simulink model "rgb_gauss_sobel_64bit_full"  (R2022a)
settings: Solver=VariableStepAuto  StartTime=0.0  StopTime=10.0  RelTol=1e-3
values from neighbouring files (symbols this model uses):
  blueMax = 255    [setup.m]
  blueMin = 75    [setup.m]
  greenMax = 255    [setup.m]
  greenMin = 75    [setup.m]
  R = 752    [setup.m]
  redMax = 255    [setup.m]
  redMin = 75    [setup.m]
undefined symbols (not defined in the file or in its folder): gray
libraries: hdlsllib x64, visionhdlio x6, visionsources x2
settings Model: PacingRate=1000  Creator=cxc1831  LastModifiedBy=calvi
settings OptimizationCC: BlockReduction=off  ConditionallyExecuteInputs=off

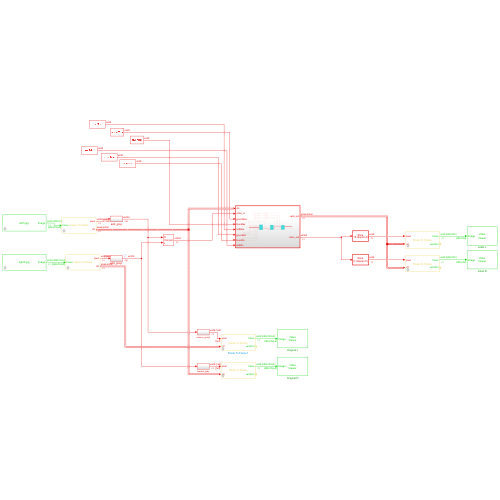
[thumbnail: Simulink's stored preview of the top-level diagram]
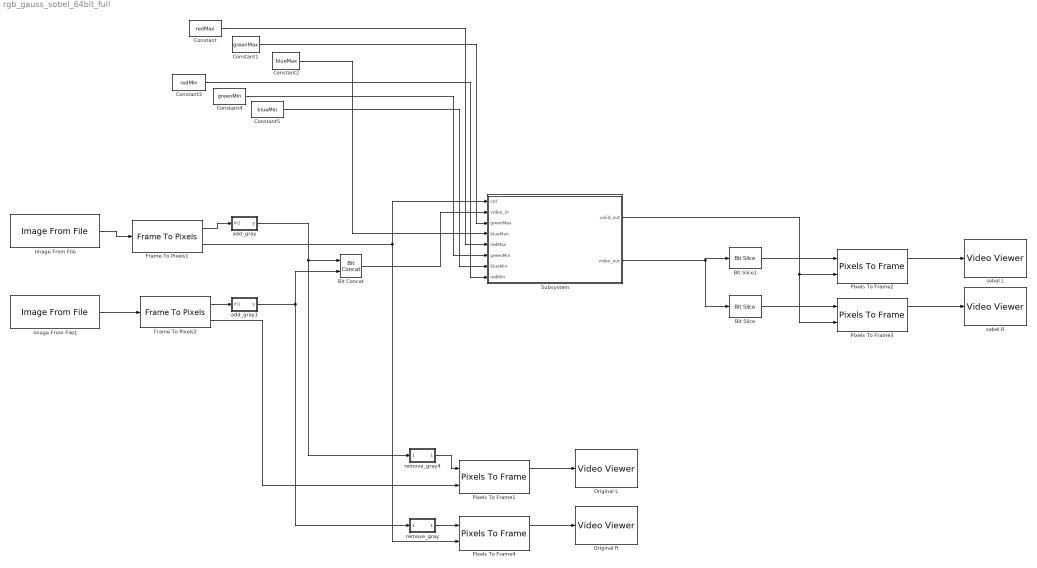
== system rgb_gauss_sobel_64bit_full ==
  Bit Concat : hdlsllib/Logic and Bit Operations/Bit Concat  numInputs=2
  Bit Slice : hdlsllib/Logic and Bit Operations/Bit Slice  lidx=7  ridx=0
      settings: SourceProductBaseCode=SL
  Bit Slice1 : hdlsllib/Logic and Bit Operations/Bit Slice  lidx=15  ridx=8
      settings: SourceProductBaseCode=SL
  Constant : Constant  Value=redMax  OutDataTypeStr=uint8  SampleTime=-1
  Constant1 : Constant  Value=greenMax  OutDataTypeStr=uint8  SampleTime=-1
  Constant2 : Constant  Value=blueMax  OutDataTypeStr=uint8  SampleTime=-1
  Constant3 : Constant  Value=redMin  OutDataTypeStr=uint8  SampleTime=-1  LockScale=on
  Constant4 : Constant  Value=greenMin  OutDataTypeStr=uint8  SampleTime=-1  LockScale=on
  Constant5 : Constant  Value=blueMin  OutDataTypeStr=uint8  SampleTime=-1  LockScale=on
  Frame To Pixels1 : visionhdlio/Frame To Pixels  NumComponents=3  NumPixels=1  VideoFormat=Custom  ActivePixelsPerLine=R  ActiveVideoLines=C  TotalPixelsPerLine=R  TotalVideoLines=C  StartingActiveLine=1  FrontPorch=0  SampleTime=0  VideoFormatCache=Custom  ActivePixelsPerLineCache=R  ActiveVideoLinesCache=C  TotalPixelsPerLineCache=R  TotalVideoLinesCache=C  StartingActiveLineCache=1  FrontPorchCache=0
      settings: SourceProductBaseCode=VT
  Frame To Pixels2 : visionhdlio/Frame To Pixels  NumComponents=3  NumPixels=1  VideoFormat=Custom  ActivePixelsPerLine=R  ActiveVideoLines=C  TotalPixelsPerLine=R  TotalVideoLines=C  StartingActiveLine=1  FrontPorch=0  SampleTime=0  VideoFormatCache=Custom  ActivePixelsPerLineCache=R  ActiveVideoLinesCache=C  TotalPixelsPerLineCache=R  TotalVideoLinesCache=C  StartingActiveLineCache=1  FrontPorchCache=0
      settings: SourceProductBaseCode=VT
  Image From File : visionsources/Image From File  Tag=vipblks_nd  FileName=C:\Projects\ipcore_integration\left3.jpg  Ts=1  imagePorts=One multidimensional signal  OutPortLabels=R|G|B  ImageDataType=Inherit from input image  sdImageDataType=uint(8)  Signed=on  WordLength=16  FractionLengthMode=User-defined  FractionLength=15
  Image From File1 : visionsources/Image From File  Tag=vipblks_nd  FileName=C:\Projects\ipcore_integration\right3.jpg  Ts=1  imagePorts=One multidimensional signal  OutPortLabels=R|G|B  ImageDataType=Inherit from input image  sdImageDataType=uint(8)  Signed=on  WordLength=16  FractionLengthMode=User-defined  FractionLength=15
  Original L : VideoViewer  colormapValue=gray(256)  FigPos=[1016 1123 562 322]
  Original R : VideoViewer  colormapValue=gray(256)  FigPos=[1046 1109 485 298]
  Pixels To Frame1 : visionhdlio/Pixels To Frame  NumComponents=3  NumPixels=1  VideoFormat=Custom  ActivePixelsPerLine=R  ActiveVideoLines=C  TotalPixelsPerLine=R  TotalVideoLines=C  VideoFormatCache=Custom  ActivePixelsPerLineCache=R  ActiveVideoLinesCache=C  TotalPixelsPerLineCache=R  TotalVideoLinesCache=C
      settings: SourceProductBaseCode=VT
  Pixels To Frame2 : visionhdlio/Pixels To Frame  NumComponents=1  NumPixels=1  VideoFormat=Custom  ActivePixelsPerLine=R  ActiveVideoLines=C  TotalPixelsPerLine=R  TotalVideoLines=C  VideoFormatCache=Custom  ActivePixelsPerLineCache=R  ActiveVideoLinesCache=C  TotalPixelsPerLineCache=R  TotalVideoLinesCache=C
      settings: SourceProductBaseCode=VT
  Pixels To Frame3 : visionhdlio/Pixels To Frame  NumComponents=1  NumPixels=1  VideoFormat=Custom  ActivePixelsPerLine=R  ActiveVideoLines=C  TotalPixelsPerLine=R  TotalVideoLines=C  VideoFormatCache=Custom  ActivePixelsPerLineCache=R  ActiveVideoLinesCache=C  TotalPixelsPerLineCache=R  TotalVideoLinesCache=C
      settings: SourceProductBaseCode=VT
  Pixels To Frame4 : visionhdlio/Pixels To Frame  NumComponents=3  NumPixels=1  VideoFormat=Custom  ActivePixelsPerLine=R  ActiveVideoLines=C  TotalPixelsPerLine=R  TotalVideoLines=C  VideoFormatCache=Custom  ActivePixelsPerLineCache=R  ActiveVideoLinesCache=C  TotalPixelsPerLineCache=R  TotalVideoLinesCache=C
      settings: SourceProductBaseCode=VT
  Subsystem : Subsystem  TreatAsAtomicUnit=on
  add_gray : Subsystem
  add_gray1 : Subsystem
  remove_gray : Subsystem
  remove_gray4 : Subsystem
  sobel L : VideoViewer  colormapValue=gray(256)  FigPos=[1 1398 2560 1298]
  sobel R : VideoViewer  colormapValue=gray(256)  FigPos=[1 1398 2560 1298]
  wires:
  Frame To Pixels2/2 -> Pixels To Frame1/2
  remove_gray4/1(RGBVector) -> Pixels To Frame1/1
  add_gray/1(y) -> remove_gray4/1(RGB), Bit Concat/1
  Image From File1/1 -> Frame To Pixels2/1
  remove_gray/1(RGBVector) -> Pixels To Frame4/1
  Frame To Pixels1/2 -> Subsystem/1(ctrl), Pixels To Frame4/2
  add_gray1/1(y) -> remove_gray/1(RGB), Bit Concat/2
  Image From File/1 -> Frame To Pixels1/1
  Frame To Pixels1/1 -> add_gray/1(In1)
  Frame To Pixels2/1 -> add_gray1/1(In1)
  Pixels To Frame1/1 -> Original L/1
  Pixels To Frame4/1 -> Original R/1
  Pixels To Frame2/1 -> sobel L/1
  Pixels To Frame3/1 -> sobel R/1
  Bit Slice/1 -> Pixels To Frame3/1
  Bit Slice1/1 -> Pixels To Frame2/1
  Bit Concat/1 -> Subsystem/2(video_in)
  Subsystem/2(video_out) -> Bit Slice1/1, Bit Slice/1
  Subsystem/1(valid_out) -> Pixels To Frame3/2, Pixels To Frame2/2
  Constant1/1 -> Subsystem/3(greenMax)
  Constant/1 -> Subsystem/5(redMax)
  Constant2/1 -> Subsystem/4(blueMax)
  Constant3/1 -> Subsystem/8(redMin)
  Constant4/1 -> Subsystem/6(greenMin)
  Constant5/1 -> Subsystem/7(blueMin)

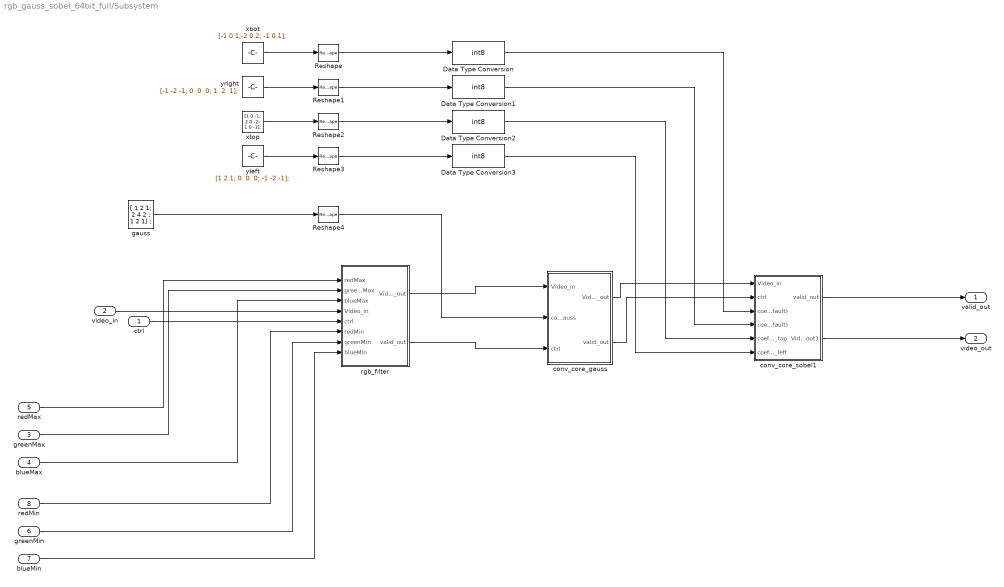
== system rgb_gauss_sobel_64bit_full/Subsystem ==
  ctrl : Inport
  video_in : Inport  Port=2
  greenMax : Inport  Port=3
  blueMax : Inport  Port=4
  redMax : Inport  Port=5
  greenMin : Inport  Port=6
  blueMin : Inport  Port=7
  redMin : Inport  Port=8
  Data Type Conversion{,1..3} (4 alike) : DataTypeConversion  OutDataTypeStr=int8  SaturateOnIntegerOverflow=off  RndMeth=Floor
  Reshape{,1..4} (5 alike) : Reshape
  conv_core_gauss : Subsystem  TreatAsAtomicUnit=on
  conv_core_sobel1 : Subsystem  TreatAsAtomicUnit=on
  gauss : Constant  Value=|  VectorParams1D=off  OutDataTypeStr=uint8  SampleTime=-1  LockScale=on
      | [ 1  2  1;  2   4   2 ;  1  2  1]
      | ;
  rgb_filter : Subsystem  TreatAsAtomicUnit=on
  xbot : Constant  Value=|  VectorParams1D=off  OutDataTypeStr=int8  SampleTime=-1
      | [-1 0 1;-2 0 2;
      | -1 0 1];
  xtop : Constant  Value=|  VectorParams1D=off  OutDataTypeStr=int8  SampleTime=-1
      | [1 0 -1; 2 0 -2;
      | 1 0 -1];
  yleft : Constant  Value="[1 2 1; 0  0  0; -1 -2 -1];"  VectorParams1D=off  OutDataTypeStr=int8  SampleTime=-1
  yright : Constant  Value=|  VectorParams1D=off  OutDataTypeStr=int8  SampleTime=-1
      | [-1 -2 -1;
      | 0  0  0; 1  2  1];
  valid_out : Outport
  video_out : Outport  Port=2
  wires:
  xtop/1 -> Reshape2/1
  yleft/1 -> Reshape3/1
  conv_core_sobel1/2(Video_out1) -> video_out/1
  xbot/1 -> Reshape/1
  yright/1 -> Reshape1/1
  conv_core_sobel1/1(valid_out) -> valid_out/1
  Reshape/1 -> Data Type Conversion/1
  Reshape1/1 -> Data Type Conversion1/1
  Reshape2/1 -> Data Type Conversion2/1
  Reshape3/1 -> Data Type Conversion3/1
  Data Type Conversion/1 -> conv_core_sobel1/3(coeffsX_bot(default))
  Data Type Conversion1/1 -> conv_core_sobel1/4(coeffsY_right(default))
  Data Type Conversion2/1 -> conv_core_sobel1/5(coeffsX_top)
  Data Type Conversion3/1 -> conv_core_sobel1/6(coeffsY_left)
  Reshape4/1 -> conv_core_gauss/2(coeffsGauss)
  gauss/1 -> Reshape4/1
  greenMin/1 -> rgb_filter/7(greenMin)
  redMax/1 -> rgb_filter/1(redMax)
  redMin/1 -> rgb_filter/6(redMin)
  greenMax/1 -> rgb_filter/2(greenMax)
  blueMax/1 -> rgb_filter/3(blueMax)
  blueMin/1 -> rgb_filter/8(blueMin)
  ctrl/1 -> rgb_filter/5(ctrl)
  video_in/1 -> rgb_filter/4(Video_in)
  rgb_filter/1(Video_out) -> conv_core_gauss/1(Video_in)
  rgb_filter/2(valid_out) -> conv_core_gauss/3(ctrl)
  conv_core_gauss/1(Video_out) -> conv_core_sobel1/1(Video_in)
  conv_core_gauss/2(valid_out) -> conv_core_sobel1/2(ctrl)

== system rgb_gauss_sobel_64bit_full/add_gray ==
  note: Grayscale = (R * 0.25) + (G * 0.5) + (B * 0.125)
  In1 : Inport
  Bit Concat : hdlsllib/Logic and Bit Operations/Bit Concat  numInputs=4
  Demux : Demux  Outputs=3
  Shift Arithmetic3 : ArithShift  BitShiftNumber=1  BitShiftDirection=Right
  Shift Arithmetic4 : ArithShift  BitShiftNumber=2  BitShiftDirection=Right
  Shift Arithmetic5 : ArithShift  BitShiftNumber=3  BitShiftDirection=Right
  Sum : Sum  Inputs=+++  OutDataTypeStr=uint8
  y : Outport
  wires:
  Bit Concat/1 -> y/1
  In1/1 -> Demux/1
  Demux/2 -> Shift Arithmetic3/1, Bit Concat/3
  Demux/1 -> Shift Arithmetic4/1, Bit Concat/2
  Demux/3 -> Shift Arithmetic5/1, Bit Concat/4
  Sum/1 -> Bit Concat/1
  Shift Arithmetic4/1 -> Sum/1
  Shift Arithmetic3/1 -> Sum/2
  Shift Arithmetic5/1 -> Sum/3

== system rgb_gauss_sobel_64bit_full/add_gray1 ==
  note: Grayscale = (R * 0.25) + (G * 0.5) + (B * 0.125)
  In1 : Inport
  Bit Concat : hdlsllib/Logic and Bit Operations/Bit Concat  numInputs=4
  Demux : Demux  Outputs=3
  Shift Arithmetic3 : ArithShift  BitShiftNumber=1  BitShiftDirection=Right
  Shift Arithmetic4 : ArithShift  BitShiftNumber=2  BitShiftDirection=Right
  Shift Arithmetic5 : ArithShift  BitShiftNumber=3  BitShiftDirection=Right
  Sum : Sum  Inputs=+++  OutDataTypeStr=uint8
  y : Outport
  wires:
  Bit Concat/1 -> y/1
  In1/1 -> Demux/1
  Demux/2 -> Shift Arithmetic3/1, Bit Concat/3
  Demux/1 -> Shift Arithmetic4/1, Bit Concat/2
  Demux/3 -> Shift Arithmetic5/1, Bit Concat/4
  Sum/1 -> Bit Concat/1
  Shift Arithmetic4/1 -> Sum/1
  Shift Arithmetic3/1 -> Sum/2
  Shift Arithmetic5/1 -> Sum/3

== system rgb_gauss_sobel_64bit_full/remove_gray ==
  note: RGB represented in
      | 32'hFFRRGGBB
  RGB : Inport
  Bit Slice : hdlsllib/Logic and Bit Operations/Bit Slice  lidx=23  ridx=16
      settings: SourceProductBaseCode=SL
  Bit Slice1 : hdlsllib/Logic and Bit Operations/Bit Slice  lidx=15  ridx=8
      settings: SourceProductBaseCode=SL
  Bit Slice2 : hdlsllib/Logic and Bit Operations/Bit Slice  lidx=7  ridx=0
      settings: SourceProductBaseCode=SL
  Mux : Mux  Inputs=3
  Signal Specification : SignalSpecification
  Transpose : Math  Operator=transpose  SignedPower=on
  RGBVector : Outport  VectorParamsAs1DForOutWhenUnconnected=off
  wires:
  Signal Specification/1 -> RGBVector/1
  Transpose/1 -> Signal Specification/1
  RGB/1 -> Bit Slice/1, Bit Slice1/1, Bit Slice2/1
  Bit Slice1/1 -> Mux/2
  Bit Slice2/1 -> Mux/3
  Bit Slice/1 -> Mux/1
  Mux/1 -> Transpose/1

== system rgb_gauss_sobel_64bit_full/remove_gray4 ==
  note: RGB represented in
      | 32'hFFRRGGBB
  RGB : Inport
  Bit Slice : hdlsllib/Logic and Bit Operations/Bit Slice  lidx=23  ridx=16
      settings: SourceProductBaseCode=SL
  Bit Slice1 : hdlsllib/Logic and Bit Operations/Bit Slice  lidx=15  ridx=8
      settings: SourceProductBaseCode=SL
  Bit Slice2 : hdlsllib/Logic and Bit Operations/Bit Slice  lidx=7  ridx=0
      settings: SourceProductBaseCode=SL
  Mux : Mux  Inputs=3
  Signal Specification : SignalSpecification
  Transpose : Math  Operator=transpose  SignedPower=on
  RGBVector : Outport  VectorParamsAs1DForOutWhenUnconnected=off
  wires:
  Signal Specification/1 -> RGBVector/1
  Transpose/1 -> Signal Specification/1
  RGB/1 -> Bit Slice/1, Bit Slice1/1, Bit Slice2/1
  Bit Slice1/1 -> Mux/2
  Bit Slice2/1 -> Mux/3
  Bit Slice/1 -> Mux/1
  Mux/1 -> Transpose/1

== system rgb_gauss_sobel_64bit_full/Subsystem/conv_core_gauss ==
  Video_in : Inport
  coeffsGauss : Inport  Port=2
  ctrl : Inport  Port=3
  Bus Selector : BusSelector  OutputSignals=valid
  Delay1 : Delay  InitialCondition=0
  Subsystem1 : Subsystem
  Video_out : Outport  VectorParamsAs1DForOutWhenUnconnected=off
  valid_out : Outport  Port=2  VectorParamsAs1DForOutWhenUnconnected=off
  wires:
  Video_in/1 -> Subsystem1/1(VideoIn)
  ctrl/1 -> Bus Selector/1, Delay1/1
  Bus Selector/1 -> Subsystem1/Enable  "<valid>"
  Subsystem1/1(Video_out) -> Video_out/1
  Delay1/1 -> valid_out/1
  coeffsGauss/1 -> Subsystem1/2(coeffsGauss)

== system rgb_gauss_sobel_64bit_full/Subsystem/conv_core_sobel1 ==
  Video_in : Inport
  ctrl : Inport  Port=2
  coeffsX_bot(default) : Inport  Port=3
  coeffsY_right(default) : Inport  Port=4
  coeffsX_top : Inport  Port=5
  coeffsY_left : Inport  Port=6
  Bit Concat1 : hdlsllib/Logic and Bit Operations/Bit Concat  numInputs=2
  Bus Selector : BusSelector  OutputSignals=valid
  Delay1 : Delay  InitialCondition=0
  Subsystem1 : Subsystem
  valid_out : Outport  VectorParamsAs1DForOutWhenUnconnected=off
  Video_out1 : Outport  Port=2  VectorParamsAs1DForOutWhenUnconnected=off
  wires:
  Video_in/1 -> Subsystem1/1(vidIn)
  ctrl/1 -> Bus Selector/1, Subsystem1/4(ctrl), Delay1/1
  Bus Selector/1 -> Subsystem1/Enable  "<valid>"
  Delay1/1 -> valid_out/1
  coeffsY_right(default)/1 -> Subsystem1/3(coeffsY_bot(default))
  coeffsX_bot(default)/1 -> Subsystem1/2(coeffsX_bot(default))
  Bit Concat1/1 -> Video_out1/1
  Subsystem1/1(sobel R) -> Bit Concat1/2
  Subsystem1/2(sobel L) -> Bit Concat1/1
  coeffsX_top/1 -> Subsystem1/5(coeffsX_Top)
  coeffsY_left/1 -> Subsystem1/6(coeffsY_Left)

== system rgb_gauss_sobel_64bit_full/Subsystem/rgb_filter ==
  redMax : Inport
  greenMax : Inport  Port=2
  blueMax : Inport  Port=3
  Video_in : Inport  Port=4
  ctrl : Inport  Port=5
  redMin : Inport  Port=6  OutDataTypeStr=uint8
  greenMin : Inport  Port=7  OutDataTypeStr=uint8
  blueMin : Inport  Port=8  OutDataTypeStr=uint8
  Bit Concat1 : hdlsllib/Logic and Bit Operations/Bit Concat  numInputs=2
  Bus Selector : BusSelector  OutputSignals=valid
  Delay1 : Delay  DelayLength=1  InitialCondition=0
  Subsystem1 : Subsystem
  Video_out : Outport  VectorParamsAs1DForOutWhenUnconnected=off
  valid_out : Outport  Port=2  VectorParamsAs1DForOutWhenUnconnected=off
  wires:
  Video_in/1 -> Subsystem1/1(In2)
  ctrl/1 -> Bus Selector/1, Delay1/1
  Bus Selector/1 -> Subsystem1/Enable  "<valid>"
  redMax/1 -> Subsystem1/2(redmax)
  Delay1/1 -> valid_out/1
  greenMax/1 -> Subsystem1/3(greenmax)
  blueMax/1 -> Subsystem1/4(bluemax)
  Bit Concat1/1 -> Video_out/1
  redMin/1 -> Subsystem1/5(redMin)
  Subsystem1/2(Video_outRight) -> Bit Concat1/2
  Subsystem1/1(Video_outLeft) -> Bit Concat1/1
  greenMin/1 -> Subsystem1/6(greenMin)
  blueMin/1 -> Subsystem1/7(blueMin)

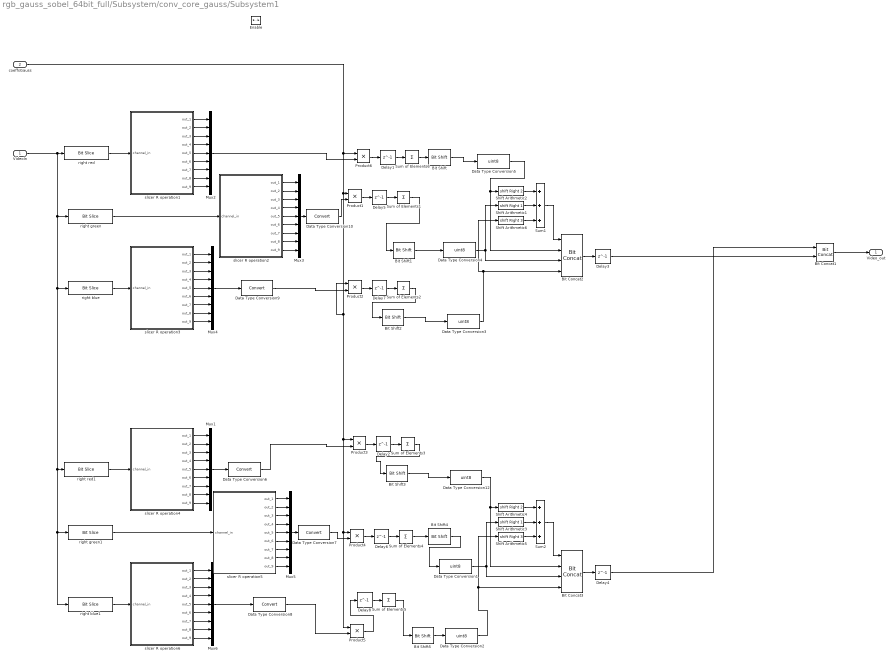
== system rgb_gauss_sobel_64bit_full/Subsystem/conv_core_gauss/Subsystem1 ==
  VideoIn : Inport
  coeffsGauss : Inport  Port=2
  Enable : EnablePort
  Bit Concat1 : hdlsllib/Logic and Bit Operations/Bit Concat  numInputs=2
  Bit Concat2 : hdlsllib/Logic and Bit Operations/Bit Concat  numInputs=4
  Bit Concat3 : hdlsllib/Logic and Bit Operations/Bit Concat  numInputs=4
  Bit Shift{,1..5} (6 alike) : hdlsllib/Logic and Bit Operations/Bit Shift  mode=Shift Right Arithmetic  N=4
  Data Type Conversion{1..5,12} (6 alike) : DataTypeConversion  OutDataTypeStr=uint8  SaturateOnIntegerOverflow=off  RndMeth=Floor
  Data Type Conversion{6..10} (5 alike) : DataTypeConversion  SaturateOnIntegerOverflow=off  RndMeth=Floor
  Delay{1..8} (8 alike) : Delay  DelayLength=1  InitialCondition=0
  Mux{1..6} (6 alike) : Mux  Inputs=9
  Product{1..6} (6 alike) : Product  SaturateOnIntegerOverflow=on
  Shift Arithmetic1 : ArithShift  BitShiftNumber=1  BitShiftDirection=Right
  Shift Arithmetic2 : ArithShift  BitShiftNumber=2  BitShiftDirection=Right
  Shift Arithmetic3 : ArithShift  BitShiftNumber=1  BitShiftDirection=Right
  Shift Arithmetic4 : ArithShift  BitShiftNumber=2  BitShiftDirection=Right
  Shift Arithmetic5 : ArithShift  BitShiftNumber=3  BitShiftDirection=Right
  Shift Arithmetic6 : ArithShift  BitShiftNumber=3  BitShiftDirection=Right
  Sum of Elements{1..6} (6 alike) : Sum  Inputs=+  OutDataTypeStr=uint32  SaturateOnIntegerOverflow=on
  Sum1 : Sum  Inputs=+++  OutDataTypeStr=uint8
  Sum2 : Sum  Inputs=+++  OutDataTypeStr=uint8
  right blue : hdlsllib/Logic and Bit Operations/Bit Slice  lidx=7  ridx=0
      settings: SourceProductBaseCode=SL
  right blue1 : hdlsllib/Logic and Bit Operations/Bit Slice  lidx=39  ridx=32
      settings: SourceProductBaseCode=SL
  right green : hdlsllib/Logic and Bit Operations/Bit Slice  lidx=15  ridx=8
      settings: SourceProductBaseCode=SL
  right green1 : hdlsllib/Logic and Bit Operations/Bit Slice  lidx=47  ridx=40
      settings: SourceProductBaseCode=SL
  right red : hdlsllib/Logic and Bit Operations/Bit Slice  lidx=23  ridx=16
      settings: SourceProductBaseCode=SL
  right red1 : hdlsllib/Logic and Bit Operations/Bit Slice  lidx=55  ridx=48
      settings: SourceProductBaseCode=SL
  slicer R operation1 : Subsystem
  slicer R operation2 : Subsystem
  slicer R operation3 : Subsystem
  slicer R operation4 : Subsystem
  slicer R operation5 : Subsystem
  slicer R operation6 : Subsystem
  Video_out : Outport  InitialOutput=0  VectorParamsAs1DForOutWhenUnconnected=off
  wires:
  right red/1 -> slicer R operation1/1(channel_in)
  right green/1 -> slicer R operation2/1(channel_in)
  right blue/1 -> slicer R operation3/1(channel_in)
  slicer R operation1/4(out_4) -> Mux2/4
  slicer R operation1/9(out_9) -> Mux2/9
  slicer R operation1/7(out_7) -> Mux2/7
  slicer R operation1/1(out_1) -> Mux2/1
  slicer R operation1/5(out_5) -> Mux2/5
  slicer R operation1/6(out_6) -> Mux2/6
  slicer R operation1/3(out_3) -> Mux2/3
  slicer R operation1/8(out_8) -> Mux2/8
  slicer R operation1/2(out_2) -> Mux2/2
  slicer R operation2/4(out_4) -> Mux3/4
  slicer R operation2/9(out_9) -> Mux3/9
  slicer R operation2/7(out_7) -> Mux3/7
  slicer R operation2/1(out_1) -> Mux3/1
  slicer R operation2/5(out_5) -> Mux3/5
  slicer R operation2/6(out_6) -> Mux3/6
  slicer R operation2/3(out_3) -> Mux3/3
  slicer R operation2/8(out_8) -> Mux3/8
  slicer R operation2/2(out_2) -> Mux3/2
  slicer R operation3/4(out_4) -> Mux4/4
  slicer R operation3/9(out_9) -> Mux4/9
  slicer R operation3/7(out_7) -> Mux4/7
  slicer R operation3/1(out_1) -> Mux4/1
  slicer R operation3/5(out_5) -> Mux4/5
  slicer R operation3/6(out_6) -> Mux4/6
  slicer R operation3/3(out_3) -> Mux4/3
  slicer R operation3/8(out_8) -> Mux4/8
  slicer R operation3/2(out_2) -> Mux4/2
  Product1/1 -> Delay5/1
  Mux3/1 -> Data Type Conversion10/1
  Mux4/1 -> Data Type Conversion9/1
  Data Type Conversion3/1 -> Shift Arithmetic6/1, Bit Concat2/4
  Sum of Elements1/1 -> Bit Shift1/1
  Data Type Conversion5/1 -> Bit Concat2/2, Shift Arithmetic2/1
  Bit Concat2/1 -> Delay3/1
  Shift Arithmetic1/1 -> Sum1/2
  Shift Arithmetic2/1 -> Sum1/1
  Shift Arithmetic6/1 -> Sum1/3
  Sum1/1 -> Bit Concat2/1
  Bit Concat1/1 -> Video_out/1
  Sum2/1 -> Bit Concat3/1
  right green1/1 -> slicer R operation5/1(channel_in)
  Shift Arithmetic4/1 -> Sum2/1
  Bit Concat3/1 -> Delay4/1
  slicer R operation4/5(out_5) -> Mux1/5
  Mux6/1 -> Data Type Conversion8/1
  Data Type Conversion12/1 -> Bit Concat3/2, Shift Arithmetic4/1
  slicer R operation6/1(out_1) -> Mux6/1
  slicer R operation4/9(out_9) -> Mux1/9
  slicer R operation6/3(out_3) -> Mux6/3
  slicer R operation6/5(out_5) -> Mux6/5
  Data Type Conversion2/1 -> Shift Arithmetic5/1, Bit Concat3/4
  slicer R operation6/9(out_9) -> Mux6/9
  slicer R operation6/8(out_8) -> Mux6/8
  slicer R operation6/4(out_4) -> Mux6/4
  right red1/1 -> slicer R operation4/1(channel_in)
  slicer R operation5/2(out_2) -> Mux5/2
  slicer R operation5/5(out_5) -> Mux5/5
  slicer R operation6/6(out_6) -> Mux6/6
  Mux1/1 -> Data Type Conversion6/1
  slicer R operation5/4(out_4) -> Mux5/4
  slicer R operation5/7(out_7) -> Mux5/7
  slicer R operation5/6(out_6) -> Mux5/6
  coeffsGauss/1 -> Product6/1, Product2/1, Product5/1, Product4/1, Product3/1, Product1/1
  slicer R operation4/7(out_7) -> Mux1/7
  slicer R operation4/3(out_3) -> Mux1/3
  slicer R operation6/7(out_7) -> Mux6/7
  slicer R operation5/3(out_3) -> Mux5/3
  Data Type Conversion1/1 -> Shift Arithmetic3/1, Bit Concat3/3
  slicer R operation5/1(out_1) -> Mux5/1
  slicer R operation5/9(out_9) -> Mux5/9
  slicer R operation4/1(out_1) -> Mux1/1
  slicer R operation4/2(out_2) -> Mux1/2
  right blue1/1 -> slicer R operation6/1(channel_in)
  slicer R operation5/8(out_8) -> Mux5/8
  Shift Arithmetic5/1 -> Sum2/3
  Shift Arithmetic3/1 -> Sum2/2
  slicer R operation6/2(out_2) -> Mux6/2
  slicer R operation4/4(out_4) -> Mux1/4
  slicer R operation4/8(out_8) -> Mux1/8
  VideoIn/1 -> right blue1/1, right green1/1, right red1/1, right blue/1, right green/1, right red/1
  slicer R operation4/6(out_6) -> Mux1/6
  Delay4/1 -> Bit Concat1/1
  Delay3/1 -> Bit Concat1/2
  Data Type Conversion6/1 -> Product3/2
  Mux5/1 -> Data Type Conversion7/1
  Data Type Conversion7/1 -> Product4/2
  Data Type Conversion8/1 -> Product5/2
  Data Type Conversion9/1 -> Product2/2
  Data Type Conversion10/1 -> Product1/2
  Mux2/1 -> Product6/2
  Bit Shift1/1 -> Data Type Conversion4/1
  Delay5/1 -> Sum of Elements1/1
  Data Type Conversion4/1 -> Bit Concat2/3, Shift Arithmetic1/1
  Bit Shift/1 -> Data Type Conversion5/1
  Sum of Elements6/1 -> Bit Shift/1
  Product6/1 -> Delay1/1
  Delay1/1 -> Sum of Elements6/1
  Bit Shift2/1 -> Data Type Conversion3/1
  Product2/1 -> Delay7/1
  Delay7/1 -> Sum of Elements2/1
  Bit Shift3/1 -> Data Type Conversion12/1
  Product3/1 -> Delay2/1
  Delay2/1 -> Sum of Elements3/1
  Bit Shift4/1 -> Data Type Conversion1/1
  Sum of Elements4/1 -> Bit Shift4/1
  Product4/1 -> Delay6/1
  Delay6/1 -> Sum of Elements4/1
  Bit Shift5/1 -> Data Type Conversion2/1
  Product5/1 -> Delay8/1
  Delay8/1 -> Sum of Elements5/1
  Sum of Elements2/1 -> Bit Shift2/1
  Sum of Elements3/1 -> Bit Shift3/1
  Sum of Elements5/1 -> Bit Shift5/1

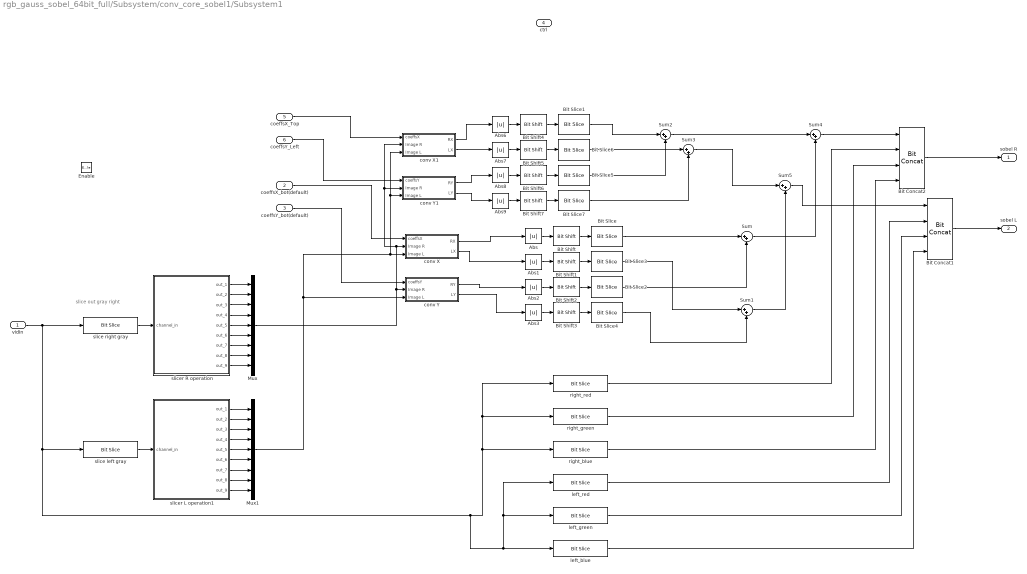
== system rgb_gauss_sobel_64bit_full/Subsystem/conv_core_sobel1/Subsystem1 ==
  note: slice out gray right
  vidIn : Inport
  coeffsX_bot(default) : Inport  Port=2
  coeffsY_bot(default) : Inport  Port=3
  ctrl : Inport  Port=4
  coeffsX_Top : Inport  Port=5
  coeffsY_Left : Inport  Port=6
  Enable : EnablePort
  Abs{,1..3,6..9} (8 alike) : Abs  SaturateOnIntegerOverflow=off
  Bit Concat1 : hdlsllib/Logic and Bit Operations/Bit Concat  numInputs=4
  Bit Concat2 : hdlsllib/Logic and Bit Operations/Bit Concat  numInputs=4
  Bit Shift{,1..7} (8 alike) : hdlsllib/Logic and Bit Operations/Bit Shift  mode=Shift Right Logical  N=1
  Bit Slice{,1..7} (8 alike) : hdlsllib/Logic and Bit Operations/Bit Slice  lidx=6  ridx=0
      settings: SourceProductBaseCode=SL
  Mux : Mux  Inputs=9
  Mux1 : Mux  Inputs=9
  Sum{,1..5} (6 alike) : Sum  Inputs=|++
  conv X : Subsystem
  conv X1 : Subsystem
  conv Y : Subsystem
  conv Y1 : Subsystem
  left_blue : hdlsllib/Logic and Bit Operations/Bit Slice  lidx=39  ridx=32
      settings: SourceProductBaseCode=SL
  left_green : hdlsllib/Logic and Bit Operations/Bit Slice  lidx=47  ridx=40
      settings: SourceProductBaseCode=SL
  left_red : hdlsllib/Logic and Bit Operations/Bit Slice  lidx=55  ridx=48
      settings: SourceProductBaseCode=SL
  right_blue : hdlsllib/Logic and Bit Operations/Bit Slice  lidx=7  ridx=0
      settings: SourceProductBaseCode=SL
  right_green : hdlsllib/Logic and Bit Operations/Bit Slice  lidx=15  ridx=8
      settings: SourceProductBaseCode=SL
  right_red : hdlsllib/Logic and Bit Operations/Bit Slice  lidx=23  ridx=16
      settings: SourceProductBaseCode=SL
  slice left gray : hdlsllib/Logic and Bit Operations/Bit Slice  lidx=63  ridx=56
      settings: SourceProductBaseCode=SL
  slice right gray : hdlsllib/Logic and Bit Operations/Bit Slice  lidx=31  ridx=24
      settings: SourceProductBaseCode=SL
  slicer L operation1 : Subsystem
  slicer R operation : Subsystem
  sobel R : Outport  InitialOutput=0
  sobel L : Outport  Port=2  InitialOutput=0
  wires:
  slicer R operation/1(out_1) -> Mux/1
  slicer R operation/9(out_9) -> Mux/9
  slicer R operation/5(out_5) -> Mux/5
  slicer R operation/7(out_7) -> Mux/7
  slicer R operation/3(out_3) -> Mux/3
  slicer R operation/6(out_6) -> Mux/6
  slicer R operation/4(out_4) -> Mux/4
  slicer R operation/2(out_2) -> Mux/2
  slicer R operation/8(out_8) -> Mux/8
  Mux/1 -> conv X/2(Image R), conv Y1/2(Image R), conv X1/2(Image R), conv Y/2(Image R)
  conv X/1(RX) -> Abs/1
  slice right gray/1 -> slicer R operation/1(channel_in)
  coeffsX_bot(default)/1 -> conv X/1(coeffsX)
  coeffsY_bot(default)/1 -> conv Y/1(coeffsY)
  slicer L operation1/9(out_9) -> Mux1/9
  slicer L operation1/8(out_8) -> Mux1/8
  slicer L operation1/6(out_6) -> Mux1/6
  slicer L operation1/5(out_5) -> Mux1/5
  slicer L operation1/3(out_3) -> Mux1/3
  slicer L operation1/2(out_2) -> Mux1/2
  slicer L operation1/7(out_7) -> Mux1/7
  slicer L operation1/4(out_4) -> Mux1/4
  slicer L operation1/1(out_1) -> Mux1/1
  slice left gray/1 -> slicer L operation1/1(channel_in)
  Mux1/1 -> conv Y/3(Image L), conv X1/3(Image L), conv Y1/3(Image L), conv X/3(Image L)
  conv Y/2(LY) -> Abs3/1
  conv X/2(LX) -> Abs1/1
  Bit Shift3/1 -> Bit Slice4/1
  Bit Shift2/1 -> Bit Slice2/1
  Bit Shift1/1 -> Bit Slice3/1
  Bit Shift/1 -> Bit Slice/1
  Bit Slice/1 -> Sum/1
  Bit Slice2/1 -> Sum/2
  Bit Slice3/1 -> Sum1/1
  Bit Slice4/1 -> Sum1/2
  conv Y/1(RY) -> Abs2/1
  Abs/1 -> Bit Shift/1
  Abs1/1 -> Bit Shift1/1
  Abs2/1 -> Bit Shift2/1
  Abs3/1 -> Bit Shift3/1
  Sum/1 -> Sum4/2
  coeffsX_Top/1 -> conv X1/1(coeffsX)
  coeffsY_Left/1 -> conv Y1/1(coeffsY)
  Bit Shift5/1 -> Bit Slice6/1
  Abs8/1 -> Bit Shift6/1
  Abs6/1 -> Bit Shift4/1
  Bit Shift6/1 -> Bit Slice5/1
  Abs9/1 -> Bit Shift7/1
  Bit Shift4/1 -> Bit Slice1/1
  Bit Shift7/1 -> Bit Slice7/1
  Abs7/1 -> Bit Shift5/1
  conv X1/1(RX) -> Abs6/1
  conv X1/2(LX) -> Abs7/1
  conv Y1/1(RY) -> Abs8/1
  conv Y1/2(LY) -> Abs9/1
  Sum2/1 -> Sum4/1
  Bit Slice1/1 -> Sum2/1
  Sum3/1 -> Sum5/1
  Sum1/1 -> Sum5/2
  Bit Slice5/1 -> Sum2/2
  Bit Slice6/1 -> Sum3/1
  Bit Slice7/1 -> Sum3/2
  vidIn/1 -> slice right gray/1, right_blue/1, right_green/1, right_red/1, left_red/1, left_green/1, left_blue/1, slice left gray/1
  Sum4/1 -> Bit Concat2/1
  Bit Concat2/1 -> sobel R/1
  right_red/1 -> Bit Concat2/2
  right_green/1 -> Bit Concat2/3
  right_blue/1 -> Bit Concat2/4
  Bit Concat1/1 -> sobel L/1
  left_blue/1 -> Bit Concat1/4
  left_green/1 -> Bit Concat1/3
  left_red/1 -> Bit Concat1/2
  Sum5/1 -> Bit Concat1/1

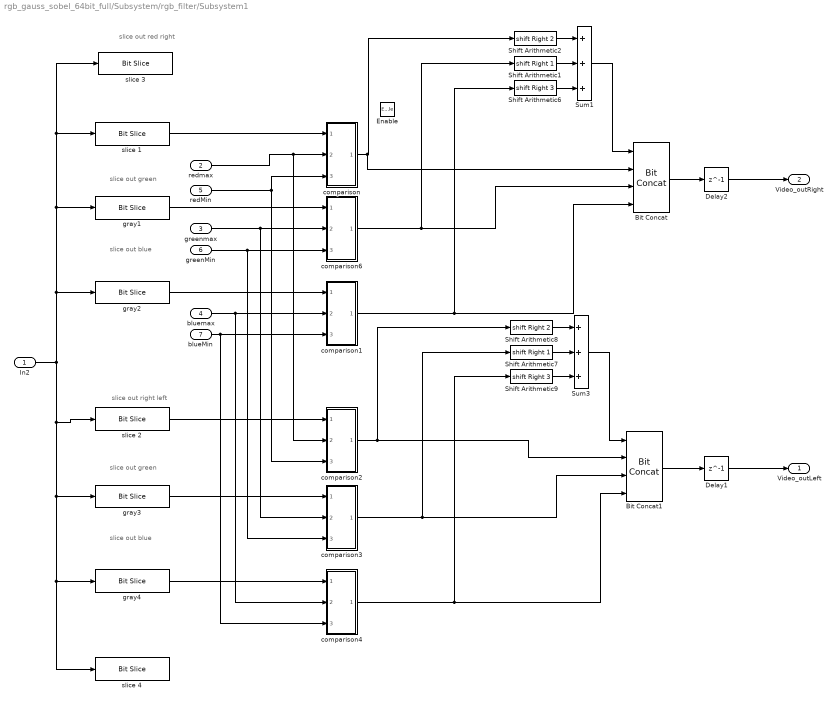
== system rgb_gauss_sobel_64bit_full/Subsystem/rgb_filter/Subsystem1 ==
  note: slice out red right
  note: slice out green
  note: slice out blue
  note: slice out blue
  note: slice out right left
  note: slice out green
  In2 : Inport
  redmax : Inport  Port=2
  greenmax : Inport  Port=3
  bluemax : Inport  Port=4
  redMin : Inport  Port=5  OutDataTypeStr=uint8
  greenMin : Inport  Port=6  OutDataTypeStr=uint8
  blueMin : Inport  Port=7  OutDataTypeStr=uint8
  Enable : EnablePort
  Bit Concat : hdlsllib/Logic and Bit Operations/Bit Concat  numInputs=4
  Bit Concat1 : hdlsllib/Logic and Bit Operations/Bit Concat  numInputs=4
  Delay1 : Delay  DelayLength=1  InitialCondition=0
  Delay2 : Delay  DelayLength=1  InitialCondition=0
  Shift Arithmetic1 : ArithShift  BitShiftNumber=1  BitShiftDirection=Right
  Shift Arithmetic2 : ArithShift  BitShiftNumber=2  BitShiftDirection=Right
  Shift Arithmetic6 : ArithShift  BitShiftNumber=3  BitShiftDirection=Right
  Shift Arithmetic7 : ArithShift  BitShiftNumber=1  BitShiftDirection=Right
  Shift Arithmetic8 : ArithShift  BitShiftNumber=2  BitShiftDirection=Right
  Shift Arithmetic9 : ArithShift  BitShiftNumber=3  BitShiftDirection=Right
  Sum1 : Sum  Inputs=+++  OutDataTypeStr=uint8
  Sum3 : Sum  Inputs=+++  OutDataTypeStr=uint8
  comparison : Subsystem
  comparison1 : Subsystem
  comparison2 : Subsystem
  comparison3 : Subsystem
  comparison4 : Subsystem
  comparison6 : Subsystem
  gray1 : hdlsllib/Logic and Bit Operations/Bit Slice  lidx=15  ridx=8
      settings: SourceProductBaseCode=SL
  gray2 : hdlsllib/Logic and Bit Operations/Bit Slice  lidx=7  ridx=0
      settings: SourceProductBaseCode=SL
  gray3 : hdlsllib/Logic and Bit Operations/Bit Slice  lidx=47  ridx=40
      settings: SourceProductBaseCode=SL
  gray4 : hdlsllib/Logic and Bit Operations/Bit Slice  lidx=39  ridx=32
      settings: SourceProductBaseCode=SL
  slice 1 : hdlsllib/Logic and Bit Operations/Bit Slice  lidx=23  ridx=16
      settings: SourceProductBaseCode=SL
  slice 2 : hdlsllib/Logic and Bit Operations/Bit Slice  lidx=55  ridx=48
      settings: SourceProductBaseCode=SL
  slice 3 : hdlsllib/Logic and Bit Operations/Bit Slice  lidx=31  ridx=24
      settings: SourceProductBaseCode=SL
  slice 4 : hdlsllib/Logic and Bit Operations/Bit Slice  lidx=63  ridx=56
      settings: SourceProductBaseCode=SL
  Video_outLeft : Outport  InitialOutput=[0]
  Video_outRight : Outport  Port=2  InitialOutput=[0]
  wires:
  Bit Concat/1 -> Delay2/1
  gray1/1 -> comparison6/1(In1)
  gray2/1 -> comparison1/1(In1)
  slice 1/1 -> comparison/1(In1)
  bluemax/1 -> comparison4/2(max), comparison1/2(max)
  comparison6/1(Out1) -> Shift Arithmetic1/1, Bit Concat/3
  comparison1/1(Out1) -> Shift Arithmetic6/1, Bit Concat/4
  redMin/1 -> comparison2/3(min), comparison/3(min)
  slice 2/1 -> comparison2/1(In1)
  greenmax/1 -> comparison3/2(max), comparison6/2(max)
  redmax/1 -> comparison2/2(max), comparison/2(max)
  In2/1 -> slice 3/1, slice 1/1, gray1/1, gray2/1, slice 4/1, gray4/1, gray3/1, slice 2/1
  gray4/1 -> comparison4/1(In1)
  gray3/1 -> comparison3/1(In1)
  Bit Concat1/1 -> Delay1/1
  blueMin/1 -> comparison4/3(min), comparison1/3(min)
  greenMin/1 -> comparison3/3(min), comparison6/3(min)
  Delay1/1 -> Video_outLeft/1
  Delay2/1 -> Video_outRight/1
  Shift Arithmetic2/1 -> Sum1/1
  Shift Arithmetic6/1 -> Sum1/3
  Shift Arithmetic1/1 -> Sum1/2
  Sum1/1 -> Bit Concat/1
  comparison/1(Out1) -> Bit Concat/2, Shift Arithmetic2/1
  comparison2/1(Out1) -> Shift Arithmetic8/1, Bit Concat1/2
  comparison4/1(Out1) -> Shift Arithmetic9/1, Bit Concat1/4
  Shift Arithmetic9/1 -> Sum3/3
  Sum3/1 -> Bit Concat1/1
  Shift Arithmetic7/1 -> Sum3/2
  Shift Arithmetic8/1 -> Sum3/1
  comparison3/1(Out1) -> Shift Arithmetic7/1, Bit Concat1/3

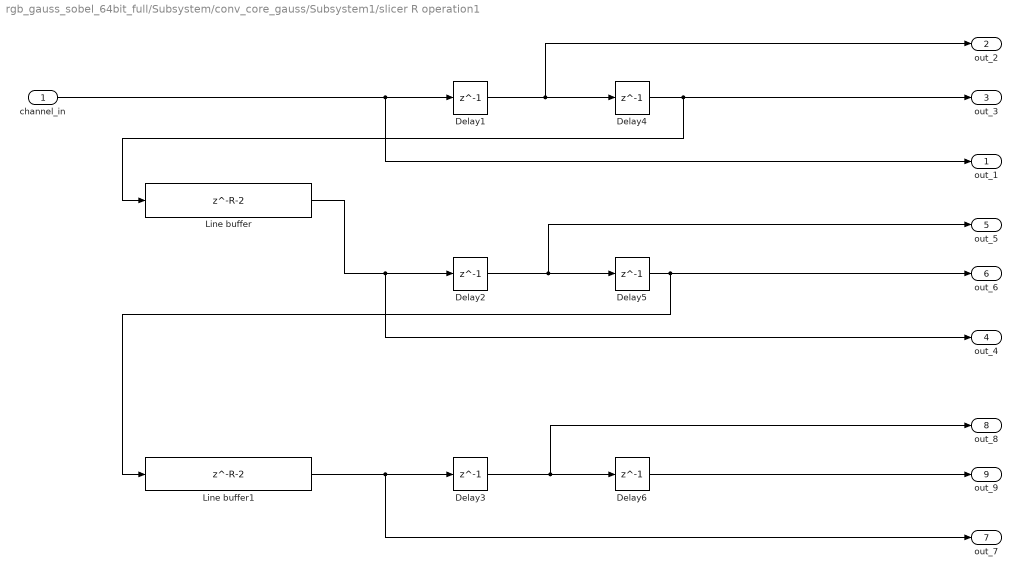
== system rgb_gauss_sobel_64bit_full/Subsystem/conv_core_gauss/Subsystem1/slicer R operation1 ==
  channel_in : Inport
  Delay{1..6} (6 alike) : Delay  DelayLength=1  InitialCondition=0
  Line buffer : Delay  DelayLength=R-2  InitialCondition=0
  Line buffer1 : Delay  DelayLength=R-2  InitialCondition=0
  out_1 : Outport  VectorParamsAs1DForOutWhenUnconnected=off
  out_2 : Outport  Port=2  VectorParamsAs1DForOutWhenUnconnected=off
  out_3 : Outport  Port=3  VectorParamsAs1DForOutWhenUnconnected=off
  out_4 : Outport  Port=4  VectorParamsAs1DForOutWhenUnconnected=off
  out_5 : Outport  Port=5  VectorParamsAs1DForOutWhenUnconnected=off
  out_6 : Outport  Port=6  VectorParamsAs1DForOutWhenUnconnected=off
  out_7 : Outport  Port=7  VectorParamsAs1DForOutWhenUnconnected=off
  out_8 : Outport  Port=8  VectorParamsAs1DForOutWhenUnconnected=off
  out_9 : Outport  Port=9  VectorParamsAs1DForOutWhenUnconnected=off
  wires:
  Delay4/1 -> Line buffer/1, out_3/1
  channel_in/1 -> out_1/1, Delay1/1
  Delay1/1 -> out_2/1, Delay4/1
  Delay3/1 -> out_8/1, Delay6/1
  Delay5/1 -> Line buffer1/1, out_6/1
  Delay6/1 -> out_9/1
  Line buffer/1 -> out_4/1, Delay2/1
  Line buffer1/1 -> out_7/1, Delay3/1
  Delay2/1 -> out_5/1, Delay5/1

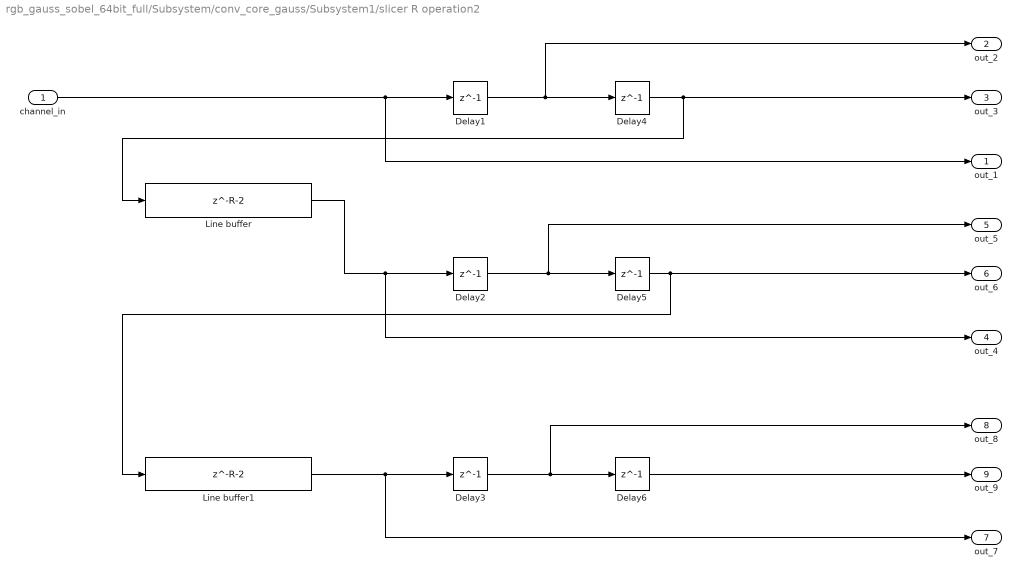
== system rgb_gauss_sobel_64bit_full/Subsystem/conv_core_gauss/Subsystem1/slicer R operation2 ==
  channel_in : Inport
  Delay{1..6} (6 alike) : Delay  DelayLength=1  InitialCondition=0
  Line buffer : Delay  DelayLength=R-2  InitialCondition=0
  Line buffer1 : Delay  DelayLength=R-2  InitialCondition=0
  out_1 : Outport  VectorParamsAs1DForOutWhenUnconnected=off
  out_2 : Outport  Port=2  VectorParamsAs1DForOutWhenUnconnected=off
  out_3 : Outport  Port=3  VectorParamsAs1DForOutWhenUnconnected=off
  out_4 : Outport  Port=4  VectorParamsAs1DForOutWhenUnconnected=off
  out_5 : Outport  Port=5  VectorParamsAs1DForOutWhenUnconnected=off
  out_6 : Outport  Port=6  VectorParamsAs1DForOutWhenUnconnected=off
  out_7 : Outport  Port=7  VectorParamsAs1DForOutWhenUnconnected=off
  out_8 : Outport  Port=8  VectorParamsAs1DForOutWhenUnconnected=off
  out_9 : Outport  Port=9  VectorParamsAs1DForOutWhenUnconnected=off
  wires:
  Delay4/1 -> Line buffer/1, out_3/1
  channel_in/1 -> out_1/1, Delay1/1
  Delay1/1 -> out_2/1, Delay4/1
  Delay3/1 -> out_8/1, Delay6/1
  Delay5/1 -> Line buffer1/1, out_6/1
  Delay6/1 -> out_9/1
  Line buffer/1 -> out_4/1, Delay2/1
  Line buffer1/1 -> out_7/1, Delay3/1
  Delay2/1 -> out_5/1, Delay5/1

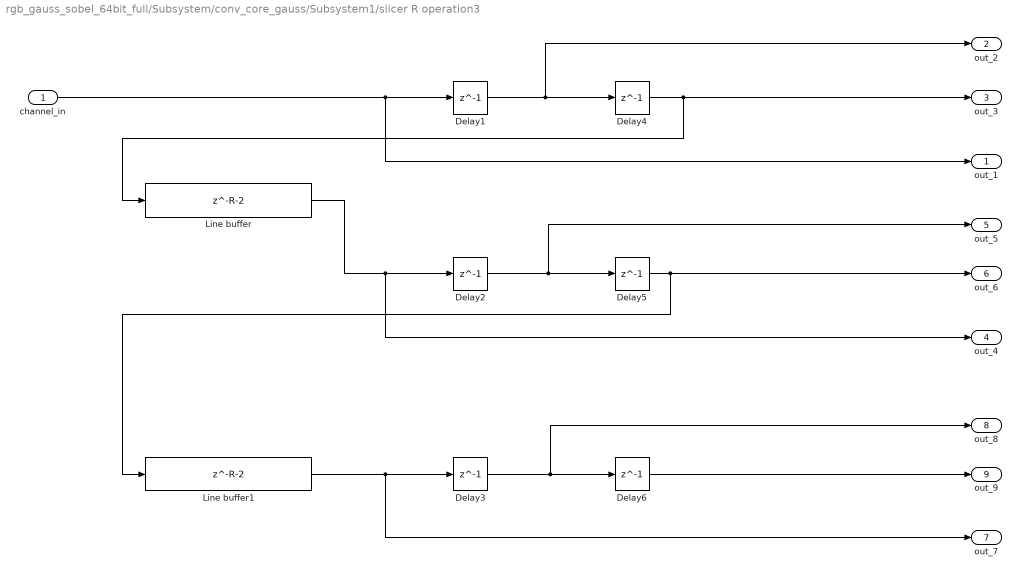
== system rgb_gauss_sobel_64bit_full/Subsystem/conv_core_gauss/Subsystem1/slicer R operation3 ==
  channel_in : Inport
  Delay{1..6} (6 alike) : Delay  DelayLength=1  InitialCondition=0
  Line buffer : Delay  DelayLength=R-2  InitialCondition=0
  Line buffer1 : Delay  DelayLength=R-2  InitialCondition=0
  out_1 : Outport  VectorParamsAs1DForOutWhenUnconnected=off
  out_2 : Outport  Port=2  VectorParamsAs1DForOutWhenUnconnected=off
  out_3 : Outport  Port=3  VectorParamsAs1DForOutWhenUnconnected=off
  out_4 : Outport  Port=4  VectorParamsAs1DForOutWhenUnconnected=off
  out_5 : Outport  Port=5  VectorParamsAs1DForOutWhenUnconnected=off
  out_6 : Outport  Port=6  VectorParamsAs1DForOutWhenUnconnected=off
  out_7 : Outport  Port=7  VectorParamsAs1DForOutWhenUnconnected=off
  out_8 : Outport  Port=8  VectorParamsAs1DForOutWhenUnconnected=off
  out_9 : Outport  Port=9  VectorParamsAs1DForOutWhenUnconnected=off
  wires:
  Delay4/1 -> Line buffer/1, out_3/1
  channel_in/1 -> out_1/1, Delay1/1
  Delay1/1 -> out_2/1, Delay4/1
  Delay3/1 -> out_8/1, Delay6/1
  Delay5/1 -> Line buffer1/1, out_6/1
  Delay6/1 -> out_9/1
  Line buffer/1 -> out_4/1, Delay2/1
  Line buffer1/1 -> out_7/1, Delay3/1
  Delay2/1 -> out_5/1, Delay5/1

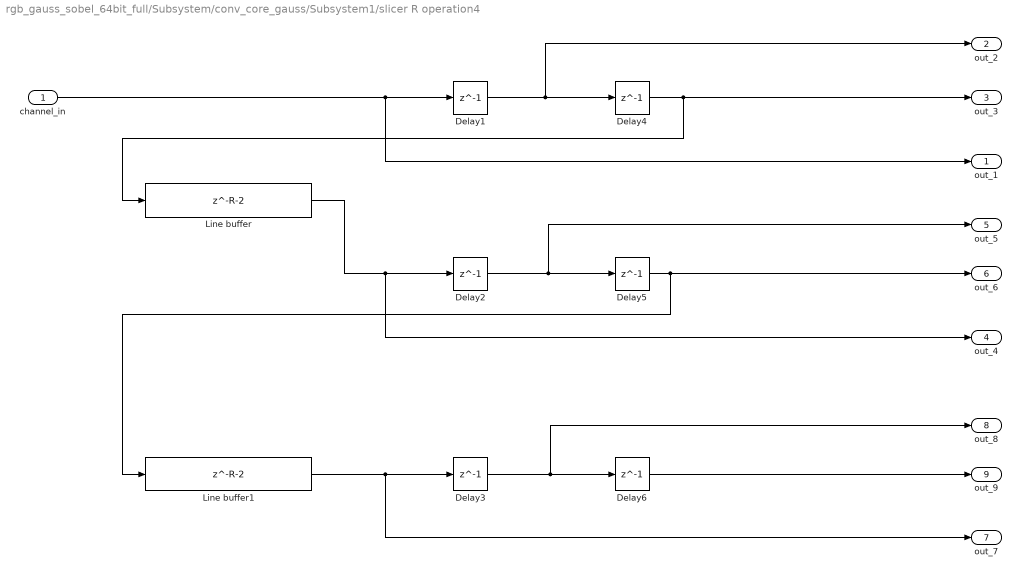
== system rgb_gauss_sobel_64bit_full/Subsystem/conv_core_gauss/Subsystem1/slicer R operation4 ==
  channel_in : Inport
  Delay{1..6} (6 alike) : Delay  DelayLength=1  InitialCondition=0
  Line buffer : Delay  DelayLength=R-2  InitialCondition=0
  Line buffer1 : Delay  DelayLength=R-2  InitialCondition=0
  out_1 : Outport  VectorParamsAs1DForOutWhenUnconnected=off
  out_2 : Outport  Port=2  VectorParamsAs1DForOutWhenUnconnected=off
  out_3 : Outport  Port=3  VectorParamsAs1DForOutWhenUnconnected=off
  out_4 : Outport  Port=4  VectorParamsAs1DForOutWhenUnconnected=off
  out_5 : Outport  Port=5  VectorParamsAs1DForOutWhenUnconnected=off
  out_6 : Outport  Port=6  VectorParamsAs1DForOutWhenUnconnected=off
  out_7 : Outport  Port=7  VectorParamsAs1DForOutWhenUnconnected=off
  out_8 : Outport  Port=8  VectorParamsAs1DForOutWhenUnconnected=off
  out_9 : Outport  Port=9  VectorParamsAs1DForOutWhenUnconnected=off
  wires:
  Delay4/1 -> Line buffer/1, out_3/1
  channel_in/1 -> out_1/1, Delay1/1
  Delay1/1 -> out_2/1, Delay4/1
  Delay3/1 -> out_8/1, Delay6/1
  Delay5/1 -> Line buffer1/1, out_6/1
  Delay6/1 -> out_9/1
  Line buffer/1 -> out_4/1, Delay2/1
  Line buffer1/1 -> out_7/1, Delay3/1
  Delay2/1 -> out_5/1, Delay5/1

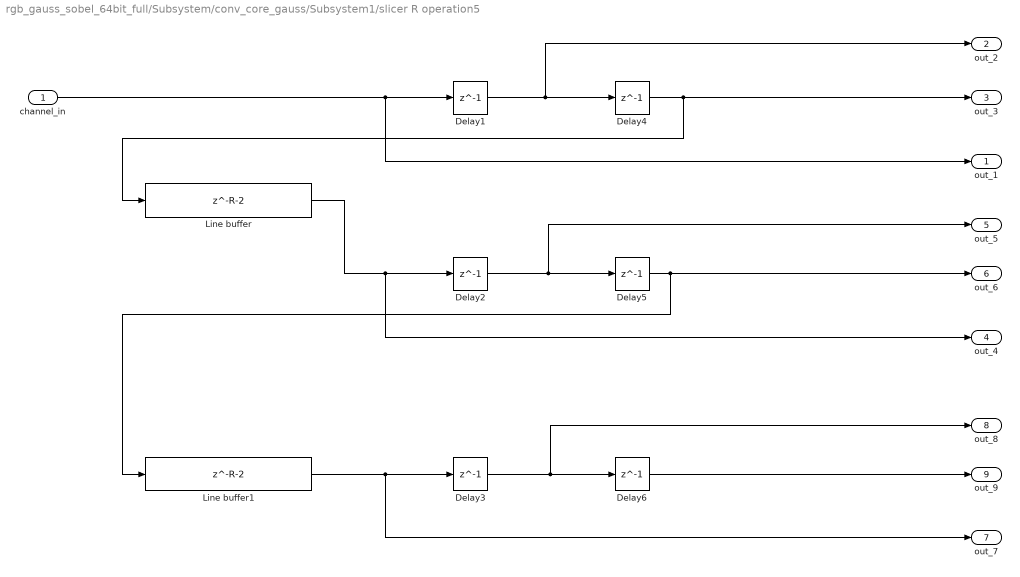
== system rgb_gauss_sobel_64bit_full/Subsystem/conv_core_gauss/Subsystem1/slicer R operation5 ==
  channel_in : Inport
  Delay{1..6} (6 alike) : Delay  DelayLength=1  InitialCondition=0
  Line buffer : Delay  DelayLength=R-2  InitialCondition=0
  Line buffer1 : Delay  DelayLength=R-2  InitialCondition=0
  out_1 : Outport  VectorParamsAs1DForOutWhenUnconnected=off
  out_2 : Outport  Port=2  VectorParamsAs1DForOutWhenUnconnected=off
  out_3 : Outport  Port=3  VectorParamsAs1DForOutWhenUnconnected=off
  out_4 : Outport  Port=4  VectorParamsAs1DForOutWhenUnconnected=off
  out_5 : Outport  Port=5  VectorParamsAs1DForOutWhenUnconnected=off
  out_6 : Outport  Port=6  VectorParamsAs1DForOutWhenUnconnected=off
  out_7 : Outport  Port=7  VectorParamsAs1DForOutWhenUnconnected=off
  out_8 : Outport  Port=8  VectorParamsAs1DForOutWhenUnconnected=off
  out_9 : Outport  Port=9  VectorParamsAs1DForOutWhenUnconnected=off
  wires:
  Delay4/1 -> Line buffer/1, out_3/1
  channel_in/1 -> out_1/1, Delay1/1
  Delay1/1 -> out_2/1, Delay4/1
  Delay3/1 -> out_8/1, Delay6/1
  Delay5/1 -> Line buffer1/1, out_6/1
  Delay6/1 -> out_9/1
  Line buffer/1 -> out_4/1, Delay2/1
  Line buffer1/1 -> out_7/1, Delay3/1
  Delay2/1 -> out_5/1, Delay5/1

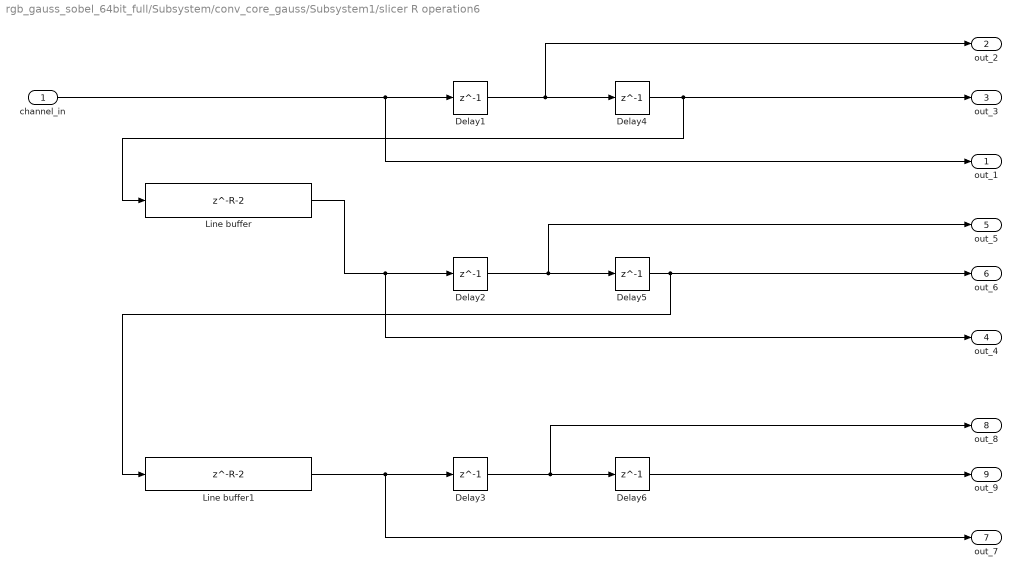
== system rgb_gauss_sobel_64bit_full/Subsystem/conv_core_gauss/Subsystem1/slicer R operation6 ==
  channel_in : Inport
  Delay{1..6} (6 alike) : Delay  DelayLength=1  InitialCondition=0
  Line buffer : Delay  DelayLength=R-2  InitialCondition=0
  Line buffer1 : Delay  DelayLength=R-2  InitialCondition=0
  out_1 : Outport  VectorParamsAs1DForOutWhenUnconnected=off
  out_2 : Outport  Port=2  VectorParamsAs1DForOutWhenUnconnected=off
  out_3 : Outport  Port=3  VectorParamsAs1DForOutWhenUnconnected=off
  out_4 : Outport  Port=4  VectorParamsAs1DForOutWhenUnconnected=off
  out_5 : Outport  Port=5  VectorParamsAs1DForOutWhenUnconnected=off
  out_6 : Outport  Port=6  VectorParamsAs1DForOutWhenUnconnected=off
  out_7 : Outport  Port=7  VectorParamsAs1DForOutWhenUnconnected=off
  out_8 : Outport  Port=8  VectorParamsAs1DForOutWhenUnconnected=off
  out_9 : Outport  Port=9  VectorParamsAs1DForOutWhenUnconnected=off
  wires:
  Delay4/1 -> Line buffer/1, out_3/1
  channel_in/1 -> out_1/1, Delay1/1
  Delay1/1 -> out_2/1, Delay4/1
  Delay3/1 -> out_8/1, Delay6/1
  Delay5/1 -> Line buffer1/1, out_6/1
  Delay6/1 -> out_9/1
  Line buffer/1 -> out_4/1, Delay2/1
  Line buffer1/1 -> out_7/1, Delay3/1
  Delay2/1 -> out_5/1, Delay5/1

== system rgb_gauss_sobel_64bit_full/Subsystem/conv_core_sobel1/Subsystem1/conv X ==
  coeffsX : Inport
  Image R : Inport  Port=2
  Image L : Inport  Port=3
  Delay{1..4} (4 alike) : Delay  DelayLength=1  InitialCondition=0
  Product : Product  SaturateOnIntegerOverflow=on
  Product1 : Product  SaturateOnIntegerOverflow=on
  Sum of Elements : Sum  Inputs=+  OutDataTypeStr=uint8  SaturateOnIntegerOverflow=on
  Sum of Elements1 : Sum  Inputs=+  OutDataTypeStr=uint8  SaturateOnIntegerOverflow=on
  RX : Outport
  LX : Outport  Port=2
  wires:
  Product/1 -> Delay1/1
  Product1/1 -> Delay2/1
  coeffsX/1 -> Product1/1, Product/2
  Image R/1 -> Product/1
  Image L/1 -> Product1/2
  Delay1/1 -> Sum of Elements/1
  Sum of Elements/1 -> Delay3/1
  Delay2/1 -> Sum of Elements1/1
  Sum of Elements1/1 -> Delay4/1
  Delay3/1 -> RX/1
  Delay4/1 -> LX/1

== system rgb_gauss_sobel_64bit_full/Subsystem/conv_core_sobel1/Subsystem1/conv X1 ==
  coeffsX : Inport
  Image R : Inport  Port=2
  Image L : Inport  Port=3
  Delay{1..4} (4 alike) : Delay  DelayLength=1  InitialCondition=0
  Display{,1..3} (4 alike) : Display
  Product : Product  SaturateOnIntegerOverflow=on
  Product1 : Product  SaturateOnIntegerOverflow=on
  Sum of Elements : Sum  Inputs=+  OutDataTypeStr=uint8  SaturateOnIntegerOverflow=on
  Sum of Elements1 : Sum  Inputs=+  OutDataTypeStr=uint8  SaturateOnIntegerOverflow=on
  RX : Outport
  LX : Outport  Port=2
  wires:
  Product/1 -> Delay1/1
  Product1/1 -> Delay2/1
  coeffsX/1 -> Product1/1, Display1/1, Product/2
  Image R/1 -> Display/1, Product/1
  Image L/1 -> Product1/2, Display2/1
  Delay1/1 -> Sum of Elements/1
  Sum of Elements/1 -> Delay3/1
  Delay2/1 -> Sum of Elements1/1
  Sum of Elements1/1 -> Display3/1, Delay4/1
  Delay3/1 -> RX/1
  Delay4/1 -> LX/1

== system rgb_gauss_sobel_64bit_full/Subsystem/conv_core_sobel1/Subsystem1/conv Y ==
  coeffsY : Inport
  Image R : Inport  Port=2
  Image L : Inport  Port=3
  Delay{1..2,4..5} (4 alike) : Delay  DelayLength=1  InitialCondition=0
  Product : Product  SaturateOnIntegerOverflow=on
  Product1 : Product  SaturateOnIntegerOverflow=on
  Sum of Elements : Sum  Inputs=+  OutDataTypeStr=uint8  SaturateOnIntegerOverflow=on
  Sum of Elements1 : Sum  Inputs=+  OutDataTypeStr=uint8  SaturateOnIntegerOverflow=on
  RY : Outport
  LY : Outport  Port=2
  wires:
  Product/1 -> Delay1/1
  Product1/1 -> Delay2/1
  coeffsY/1 -> Product1/1, Product/2
  Image R/1 -> Product/1
  Image L/1 -> Product1/2
  Delay1/1 -> Sum of Elements/1
  Sum of Elements/1 -> Delay5/1
  Delay2/1 -> Sum of Elements1/1
  Sum of Elements1/1 -> Delay4/1
  Delay5/1 -> RY/1
  Delay4/1 -> LY/1

== system rgb_gauss_sobel_64bit_full/Subsystem/conv_core_sobel1/Subsystem1/conv Y1 ==
  coeffsY : Inport
  Image R : Inport  Port=2
  Image L : Inport  Port=3
  Delay{1..2,4..5} (4 alike) : Delay  DelayLength=1  InitialCondition=0
  Product : Product  SaturateOnIntegerOverflow=on
  Product1 : Product  SaturateOnIntegerOverflow=on
  Sum of Elements : Sum  Inputs=+  OutDataTypeStr=uint8  SaturateOnIntegerOverflow=on
  Sum of Elements1 : Sum  Inputs=+  OutDataTypeStr=uint8  SaturateOnIntegerOverflow=on
  RY : Outport
  LY : Outport  Port=2
  wires:
  Product/1 -> Delay1/1
  Product1/1 -> Delay2/1
  coeffsY/1 -> Product1/1, Product/2
  Image R/1 -> Product/1
  Image L/1 -> Product1/2
  Delay1/1 -> Sum of Elements/1
  Sum of Elements/1 -> Delay5/1
  Delay2/1 -> Sum of Elements1/1
  Sum of Elements1/1 -> Delay4/1
  Delay5/1 -> RY/1
  Delay4/1 -> LY/1

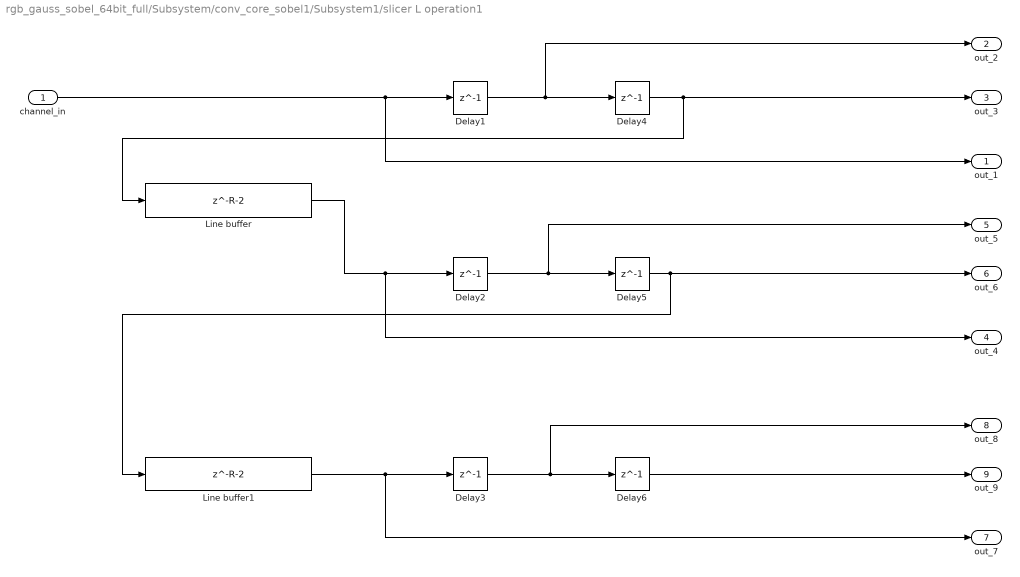
== system rgb_gauss_sobel_64bit_full/Subsystem/conv_core_sobel1/Subsystem1/slicer L operation1 ==
  channel_in : Inport
  Delay{1..6} (6 alike) : Delay  DelayLength=1  InitialCondition=0
  Line buffer : Delay  DelayLength=R-2  InitialCondition=0
  Line buffer1 : Delay  DelayLength=R-2  InitialCondition=0
  out_1 : Outport  VectorParamsAs1DForOutWhenUnconnected=off
  out_2 : Outport  Port=2  VectorParamsAs1DForOutWhenUnconnected=off
  out_3 : Outport  Port=3  VectorParamsAs1DForOutWhenUnconnected=off
  out_4 : Outport  Port=4  VectorParamsAs1DForOutWhenUnconnected=off
  out_5 : Outport  Port=5  VectorParamsAs1DForOutWhenUnconnected=off
  out_6 : Outport  Port=6  VectorParamsAs1DForOutWhenUnconnected=off
  out_7 : Outport  Port=7  VectorParamsAs1DForOutWhenUnconnected=off
  out_8 : Outport  Port=8  VectorParamsAs1DForOutWhenUnconnected=off
  out_9 : Outport  Port=9  VectorParamsAs1DForOutWhenUnconnected=off
  wires:
  Delay4/1 -> Line buffer/1, out_3/1
  channel_in/1 -> out_1/1, Delay1/1
  Delay1/1 -> out_2/1, Delay4/1
  Delay3/1 -> out_8/1, Delay6/1
  Delay5/1 -> Line buffer1/1, out_6/1
  Delay6/1 -> out_9/1
  Line buffer/1 -> out_4/1, Delay2/1
  Line buffer1/1 -> out_7/1, Delay3/1
  Delay2/1 -> out_5/1, Delay5/1

== system rgb_gauss_sobel_64bit_full/Subsystem/conv_core_sobel1/Subsystem1/slicer R operation ==
  channel_in : Inport
  Delay{1..6} (6 alike) : Delay  DelayLength=1  InitialCondition=0
  Line buffer : Delay  DelayLength=R-2  InitialCondition=0
  Line buffer1 : Delay  DelayLength=R-2  InitialCondition=0
  out_1 : Outport  VectorParamsAs1DForOutWhenUnconnected=off
  out_2 : Outport  Port=2  VectorParamsAs1DForOutWhenUnconnected=off
  out_3 : Outport  Port=3  VectorParamsAs1DForOutWhenUnconnected=off
  out_4 : Outport  Port=4  VectorParamsAs1DForOutWhenUnconnected=off
  out_5 : Outport  Port=5  VectorParamsAs1DForOutWhenUnconnected=off
  out_6 : Outport  Port=6  VectorParamsAs1DForOutWhenUnconnected=off
  out_7 : Outport  Port=7  VectorParamsAs1DForOutWhenUnconnected=off
  out_8 : Outport  Port=8  VectorParamsAs1DForOutWhenUnconnected=off
  out_9 : Outport  Port=9  VectorParamsAs1DForOutWhenUnconnected=off
  wires:
  Delay4/1 -> Line buffer/1, out_3/1
  channel_in/1 -> out_1/1, Delay1/1
  Delay1/1 -> out_2/1, Delay4/1
  Delay3/1 -> out_8/1, Delay6/1
  Delay5/1 -> Line buffer1/1, out_6/1
  Delay6/1 -> out_9/1
  Line buffer/1 -> out_4/1, Delay2/1
  Line buffer1/1 -> out_7/1, Delay3/1
  Delay2/1 -> out_5/1, Delay5/1

== system rgb_gauss_sobel_64bit_full/Subsystem/rgb_filter/Subsystem1/comparison ==
  In1 : Inport
  max : Inport  Port=2
  min : Inport  Port=3
  AND : Logic  IconShape=distinctive  AllPortsSameDT=off  OutDataTypeStr=boolean
  Constant : Constant  Value=0  OutDataTypeStr=uint8  SampleTime=-1
  Relational Operator : RelationalOperator  Operator=<=  OutDataTypeStr=boolean  RndMeth=Simplest  InputSameDT=off
  Relational Operator1 : RelationalOperator  OutDataTypeStr=boolean  RndMeth=Simplest  InputSameDT=off
  Switch : Switch  Criteria=u2 ~= 0  SaturateOnIntegerOverflow=off  InputSameDT=off
  Out1 : Outport
  wires:
  Constant/1 -> Switch/3
  In1/1 -> Relational Operator1/1, Switch/1, Relational Operator/1
  Relational Operator/1 -> AND/1
  max/1 -> Relational Operator/2
  Switch/1 -> Out1/1
  Relational Operator1/1 -> AND/2
  min/1 -> Relational Operator1/2
  AND/1 -> Switch/2

== system rgb_gauss_sobel_64bit_full/Subsystem/rgb_filter/Subsystem1/comparison1 ==
  In1 : Inport
  max : Inport  Port=2
  min : Inport  Port=3
  AND : Logic  IconShape=distinctive  AllPortsSameDT=off  OutDataTypeStr=boolean
  Constant : Constant  Value=0  OutDataTypeStr=uint8  SampleTime=-1
  Relational Operator : RelationalOperator  Operator=<=  OutDataTypeStr=boolean  RndMeth=Simplest  InputSameDT=off
  Relational Operator1 : RelationalOperator  OutDataTypeStr=boolean  RndMeth=Simplest  InputSameDT=off
  Switch : Switch  Criteria=u2 ~= 0  SaturateOnIntegerOverflow=off  InputSameDT=off
  Out1 : Outport
  wires:
  Constant/1 -> Switch/3
  In1/1 -> Relational Operator1/1, Switch/1, Relational Operator/1
  Relational Operator/1 -> AND/1
  max/1 -> Relational Operator/2
  Switch/1 -> Out1/1
  Relational Operator1/1 -> AND/2
  min/1 -> Relational Operator1/2
  AND/1 -> Switch/2

== system rgb_gauss_sobel_64bit_full/Subsystem/rgb_filter/Subsystem1/comparison2 ==
  In1 : Inport
  max : Inport  Port=2
  min : Inport  Port=3
  AND : Logic  IconShape=distinctive  AllPortsSameDT=off  OutDataTypeStr=boolean
  Constant : Constant  Value=0  OutDataTypeStr=uint8  SampleTime=-1
  Relational Operator : RelationalOperator  Operator=<=  OutDataTypeStr=boolean  RndMeth=Simplest  InputSameDT=off
  Relational Operator1 : RelationalOperator  OutDataTypeStr=boolean  RndMeth=Simplest  InputSameDT=off
  Switch : Switch  Criteria=u2 ~= 0  SaturateOnIntegerOverflow=off  InputSameDT=off
  Out1 : Outport
  wires:
  Constant/1 -> Switch/3
  In1/1 -> Relational Operator1/1, Switch/1, Relational Operator/1
  Relational Operator/1 -> AND/1
  max/1 -> Relational Operator/2
  Switch/1 -> Out1/1
  Relational Operator1/1 -> AND/2
  min/1 -> Relational Operator1/2
  AND/1 -> Switch/2

== system rgb_gauss_sobel_64bit_full/Subsystem/rgb_filter/Subsystem1/comparison3 ==
  In1 : Inport
  max : Inport  Port=2
  min : Inport  Port=3
  AND : Logic  IconShape=distinctive  AllPortsSameDT=off  OutDataTypeStr=boolean
  Constant : Constant  Value=0  OutDataTypeStr=uint8  SampleTime=-1
  Relational Operator : RelationalOperator  Operator=<=  OutDataTypeStr=boolean  RndMeth=Simplest  InputSameDT=off
  Relational Operator1 : RelationalOperator  OutDataTypeStr=boolean  RndMeth=Simplest  InputSameDT=off
  Switch : Switch  Criteria=u2 ~= 0  SaturateOnIntegerOverflow=off  InputSameDT=off
  Out1 : Outport
  wires:
  Constant/1 -> Switch/3
  In1/1 -> Relational Operator1/1, Switch/1, Relational Operator/1
  Relational Operator/1 -> AND/1
  max/1 -> Relational Operator/2
  Switch/1 -> Out1/1
  Relational Operator1/1 -> AND/2
  min/1 -> Relational Operator1/2
  AND/1 -> Switch/2

== system rgb_gauss_sobel_64bit_full/Subsystem/rgb_filter/Subsystem1/comparison4 ==
  In1 : Inport
  max : Inport  Port=2
  min : Inport  Port=3
  AND : Logic  IconShape=distinctive  AllPortsSameDT=off  OutDataTypeStr=boolean
  Constant : Constant  Value=0  OutDataTypeStr=uint8  SampleTime=-1
  Relational Operator : RelationalOperator  Operator=<=  OutDataTypeStr=boolean  RndMeth=Simplest  InputSameDT=off
  Relational Operator1 : RelationalOperator  OutDataTypeStr=boolean  RndMeth=Simplest  InputSameDT=off
  Switch : Switch  Criteria=u2 ~= 0  SaturateOnIntegerOverflow=off  InputSameDT=off
  Out1 : Outport
  wires:
  Constant/1 -> Switch/3
  In1/1 -> Relational Operator1/1, Switch/1, Relational Operator/1
  Relational Operator/1 -> AND/1
  max/1 -> Relational Operator/2
  Switch/1 -> Out1/1
  Relational Operator1/1 -> AND/2
  min/1 -> Relational Operator1/2
  AND/1 -> Switch/2

== system rgb_gauss_sobel_64bit_full/Subsystem/rgb_filter/Subsystem1/comparison6 ==
  In1 : Inport
  max : Inport  Port=2
  min : Inport  Port=3
  AND : Logic  IconShape=distinctive  AllPortsSameDT=off  OutDataTypeStr=boolean
  Constant : Constant  Value=0  OutDataTypeStr=uint8  SampleTime=-1
  Relational Operator : RelationalOperator  Operator=<=  OutDataTypeStr=boolean  RndMeth=Simplest  InputSameDT=off
  Relational Operator1 : RelationalOperator  OutDataTypeStr=boolean  RndMeth=Simplest  InputSameDT=off
  Switch : Switch  Criteria=u2 ~= 0  SaturateOnIntegerOverflow=off  InputSameDT=off
  Out1 : Outport
  wires:
  Constant/1 -> Switch/3
  In1/1 -> Relational Operator1/1, Switch/1, Relational Operator/1
  Relational Operator/1 -> AND/1
  max/1 -> Relational Operator/2
  Switch/1 -> Out1/1
  Relational Operator1/1 -> AND/2
  min/1 -> Relational Operator1/2
  AND/1 -> Switch/2
